simulink model "ModelDemopalooza"  (R2022b)
settings: Solver=FixedStepDiscrete  StartTime=0.0  StopTime=1  RelTol=1e-3  EnableMultiTasking=on
InitFcn:
  | % Initialize model
  | run(['ModelInit.m']);
  | 
  | % load library data
  | GainLibrary_data;
StartFcn:
  | % make sure all the simulated RTC requests are found
  | %RTC_SIM_OBJ.ValidateREQs();
model workspace (MAT data in the model file):
  PreampVolumeTable_Idx = Simulink.Signal
  PreampVolumeTable_Idx.DataType = 'auto'
  PreampVolumeTable_Idx.Dimensions = -1
  PreampVolumeTable_Idx.DimensionsMode = 'auto'
  PreampVolumeTable_Idx.Complexity = 'auto'
  PreampVolumeTable_Idx.SampleTime = -1
  PreampVolumeTable_Idx.SamplingMode = 'auto'
  PreampVolumeTable_Idx.InitialValue = 'uint8([0 255 255 255 255 255])'
  Range = Simulink.Signal
  Range.DataType = 'auto'
  Range.Dimensions = -1
  Range.DimensionsMode = 'auto'
  Range.Complexity = 'auto'
  Range.SampleTime = -1
  Range.SamplingMode = 'auto'
  Table_Idx = Simulink.Signal
  Table_Idx.DataType = 'auto'
  Table_Idx.Dimensions = -1
  Table_Idx.DimensionsMode = 'auto'
  Table_Idx.Complexity = 'auto'
  Table_Idx.SampleTime = -1
  Table_Idx.SamplingMode = 'auto'
undefined symbols (not defined in the file): Config, Ifir, IFIR, MedusaConfig, MuteRamper, MuteRamperBtc, numAudioIn, preAmp, Row, sys_defs, VLSConfig
libraries: FeaturePath x22, TuneVar x17, RTC x9, MedusaDelays x9, dspindex x5, TOP x5, SampleRateConverter x4, EdgePorts x2, PooliirLib x2, MedusaCaeEnable x2, FIREven x2, VLSGains x2
(part 1 of 4)
settings Model: Creator=kl13806  LastModifiedBy=sc48041
settings SolverCC: AlgebraicLoopSolver=TrustRegion  AutoInsertRateTranBlk=on
settings OptimizationCC: DefaultParameterBehavior=Inlined  DefaultUnderspecifiedDataType=single  ZeroExternalMemoryAtStartup=off  ZeroInternalMemoryAtStartup=off  MaxStackSize=2048  DifferentSizesBufferReuse=on  EfficientTunableParamExpr=on
settings DebuggingCC: InheritedTsInSrcMsg=none  MultiTaskDSMMsg=none  MultiTaskRateTransMsg=warning  ParameterPrecisionLossMsg=none  ParameterTunabilityLossMsg=error  UnconnectedInputMsg=warning  UnconnectedOutputMsg=warning  UnconnectedLineMsg=warning  BusObjectLabelMismatch=none  UnknownTsInhSupMsg=none  SFUnexpectedBacktrackingDiag=warning  SFNoUnconditionalDefaultTransitionDiag=warning  SFExecutionAtInitializationDiag=none  SFMachineParentedDataDiag=warning  ArithmeticOperatorsInVariantConditions=warning
settings HardwareCC: ProdBitPerDouble=32  ProdBitPerPointer=32  ProdBitPerSizeT=32  ProdBitPerPtrDiffT=32  ProdLargestAtomicInteger=Long  ProdLargestAtomicFloat=Double  ProdWordSize=32  ProdHWDeviceType=Qualcomm->Hexagon  TargetBitPerPointer=64  TargetBitPerSizeT=64  TargetBitPerPtrDiffT=64  TargetLargestAtomicInteger=Integer  TargetLongLongMode=on  TargetIntDivRoundTo=Zero  TargetEndianess=LittleEndian  TargetWordSize=64  TargetHWDeviceType=MATLAB Host  ProdEqTarget=off
settings ModelReferenceCC: EnableRefExpFcnMdlSchedulingChecks=on
settings SFSimCC: SimUseLocalCustomCode=off  MATLABDynamicMemAlloc=off  CustomCodeUndefinedFunction=UseInterfaceOnly
settings RTWCC: Description=Embedded Coder (host-based shared library target)  SystemTargetFile=ert_shrlib.tlc  GenCodeOnly=on  TemplateMakefile=ert_default_tmf  GenerateReport=on  RetainRTWFile=on  RTWUseLocalCustomCode=off  BuildConfiguration=Faster Runs  IncludeHyperlinkInReport=on  LaunchReport=on  GenerateTraceInfo=on  GenerateTraceReport=on  GenerateTraceReportSl=on  GenerateTraceReportSf=on  GenerateTraceReportEml=on  GenerateCodeMetricsReport=on  GenerateCodeReplacementReport=on
settings CodeAppCC: ForceParamTrailComments=on  IgnoreCustomStorageClasses=off  MaxIdLength=61  OperatorAnnotations=on  SimulinkDataObjDesc=on  SFDataObjDesc=on  MATLABFcnDesc=on  InsertBlockDesc=on  StateflowObjectComments=on  MATLABSourceComments=on
settings STFCustomTargetCC: TargetLangStandard=C99 (ISO)  CodeReplacementLibrary=Qualcomm Hexagon DSP code replacement library  ParMdlRefBuildCompliant=on  CompOptLevelCompliant=on  CombineOutputUpdateFcns=on  ERTCustomFileBanners=on  SupportNonFinite=off  SupportContinuousTime=off  SupportNonInlinedSFcns=off  RemoveResetFunc=on  SupportVariableSizeSignals=on  MATLABClassNameForMDSCustomization=Simulink.SoftwareTarget.ERTCustomization  ModelStepFunctionPrototypeControlCompliant=on  UseToolchainInfoCompliant=on  SystemTargetFile=ert_shrlib.tlc
settings ERTTargetCC: TargetLangStandard=C99 (ISO)  CodeReplacementLibrary=Qualcomm Hexagon DSP code replacement library  MultiwordLength=2048  ConcurrentExecutionCompliant=off  SupportNonFinite=off  SupportVariableSizeSignals=on  CPPClassGenCompliant=off  InlinedParameterPlacement=NonHierarchical  ERTCustomFileTemplate=example_file_process.tlc  IndentStyle=Allman  IndentSize=4
settings ConfigComp: CovMetricSettings=dw  CovSaveCumulativeToWorkspaceVar=on  CovSaveSingleToWorkspaceVar=on  CovExternalEMLEnable=off

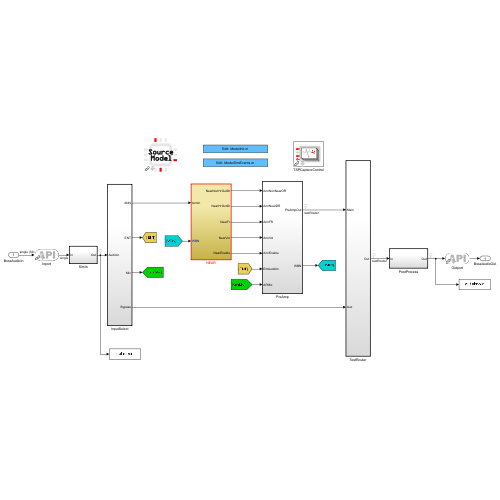
[thumbnail: Simulink's stored preview of the top-level diagram]
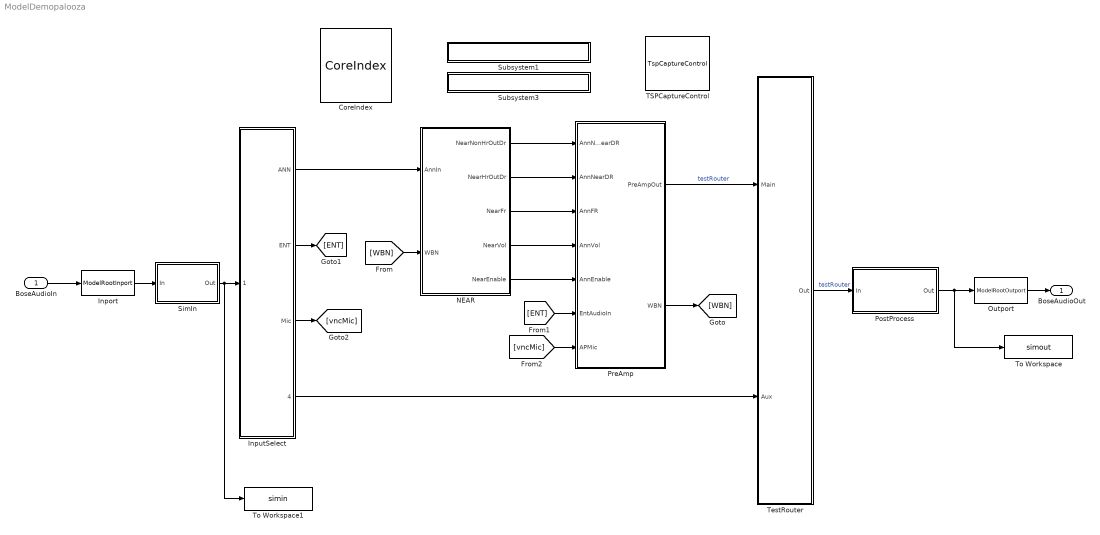
== system ModelDemopalooza ==
  BoseAudioIn : Inport  OutDataTypeStr=single  PortDimensions=[sys_defs.frameSize numAudioIn]  SampleTime=1/sys_defs.Fs * sys_defs.frameSize
  CoreIndex : FeaturePath/CoreIndex  Role=Source Model  CoreIndex=8  Config=[]  AddressingMode=Directly include core number in message identifiers (i.e. simple and static)  CrossCoreApi=None  CrossCoreAllocation=None  CrossCoreSampleTime=-1  BasePeriod=[]  TriggerInit=[-15 -776 80 -679]
      settings: SourceProductName=Bose Talaria
  Inport : EdgePorts/ModelRootInport  Config=ModelRootIn
      settings: SourceProductName=Bose Talaria
  InputSelect : Subsystem  TreatAsAtomicUnit=on
      settings: RTWSystemCode=Nonreusable function
  NEAR : Subsystem  TreatAsAtomicUnit=on
  Outport : EdgePorts/ModelRootOutport  Config=ModelRootOut
      settings: SourceProductName=Bose Talaria
  PostProcess : Subsystem  TreatAsAtomicUnit=on
  PreAmp : Subsystem  TreatAsAtomicUnit=on
  SimIn : Subsystem  TreatAsAtomicUnit=on
  Subsystem1 : Subsystem  mask{filename=Init.m}
      settings: OpenFcn=edit([ ModelRootName() get(gcbh,'filename') ]);
      mask Display: disp(['Edit: ' ModelRootName() get(gcbh,'filename')]);
  Subsystem3 : Subsystem  mask{filename=SimEvents.m}
      settings: OpenFcn=edit([ ModelRootName() get(gcbh,'filename') ]);
      mask Display: disp(['Edit: ' ModelRootName() get(gcbh,'filename')]);
  TSPCaptureControl : TSP/TspCaptureControl  TriggerInit=[415 -766 500 -694]
      settings: SourceProductName=Bose Talaria
  TestRouter : Subsystem  TreatAsAtomicUnit=on
  To Workspace : ToWorkspace  VariableName=simout  SaveFormat=Timeseries  SampleTime=-1
  To Workspace1 : ToWorkspace  VariableName=simin  SaveFormat=Timeseries  SampleTime=-1
  BoseAudioOut : Outport  VectorParamsAs1DForOutWhenUnconnected=off
  wires:
  SimIn/1(Out) -> To Workspace1/1, InputSelect/1(AudioIn)
  BoseAudioIn/1 -> Inport/1
  Inport/1 -> SimIn/1(In)
  Outport/1 -> BoseAudioOut/1
  InputSelect/1(ANN) -> NEAR/1(AnnIn)
  [WBN] -> NEAR/2(WBN)
  NEAR/5(NearEnable) -> PreAmp/5(AnnEnable)
  NEAR/4(NearVol) -> PreAmp/4(AnnVol)
  NEAR/3(NearFr) -> PreAmp/3(AnnFR)
  PreAmp/2(WBN) -> [WBN]
  NEAR/1(NearNonHrOutDr) -> PreAmp/1(AnnNonNearDR)
  NEAR/2(NearHrOutDr) -> PreAmp/2(AnnNearDR)
  InputSelect/2(ENT) -> [ENT]
  [ENT] -> PreAmp/6(EntAudioIn)
  InputSelect/3(Mic) -> [vncMic]
  [vncMic] -> PreAmp/7(APMic)
  PreAmp/1(PreAmpOut) -> TestRouter/1(Main)  "testRouter"
  TestRouter/1(Out) -> PostProcess/1(In)  "testRouter"
  PostProcess/1(Out) -> To Workspace/1, Outport/1
  InputSelect/4(Bypass) -> TestRouter/2(Aux)

== system ModelDemopalooza/InputSelect ==
  AudioIn : Inport
  FeaturePath : FeaturePath/FeaturePath  FeatureName=InputSelect  IsGroup=on  GroupNumber=0  IsModule=on  TriggerInit=[105 216 220 329]
      settings: SourceProductName=Bose Talaria
  Partition : FeaturePath/Partition  PartitionNumber=0  TriggerInit=[250 241 295 309]
      settings: SourceProductName=Bose Talaria
  Reset : Subsystem  Commented=on
  Variable Selector1 : dspindex/Variable Selector  NumInputs=1  rowsOrCols=Columns  IdxMode=Fixed  Elements=entMap  ZerOneIdxMode=One-based  errmode=Clip Index  FillMode=on  FillValues=0
  Variable Selector2 : dspindex/Variable Selector  NumInputs=1  rowsOrCols=Columns  IdxMode=Fixed  Elements=annMap  ZerOneIdxMode=One-based  errmode=Clip Index  FillMode=on  FillValues=0
  Variable Selector3 : dspindex/Variable Selector  NumInputs=1  rowsOrCols=Columns  IdxMode=Fixed  Elements=vncMic  ZerOneIdxMode=One-based  errmode=Clip Index  FillMode=on  FillValues=0
  router : Router/Router  nInRouterMask=inputSelectChanIn  nOutRouterMask=inputSelectChanOut  outputMapDefaultRouterMask=inputSelectOutputMap
  ANN : Outport
  ENT : Outport  Port=2  VectorParamsAs1DForOutWhenUnconnected=off
  Mic : Outport  Port=3
  Bypass : Outport  Port=4  VectorParamsAs1DForOutWhenUnconnected=off
  wires:
  Variable Selector1/1 -> ENT/1
  AudioIn/1 -> Bypass/1, router/1
  router/1 -> Variable Selector3/1, Variable Selector2/1, Variable Selector1/1
  Variable Selector2/1 -> ANN/1
  Variable Selector3/1 -> Mic/1

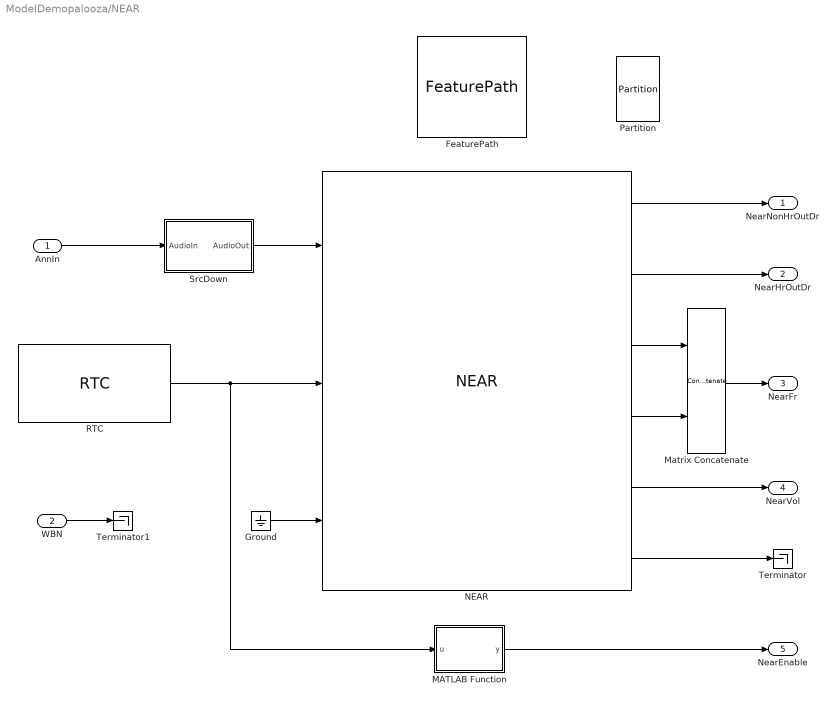
== system ModelDemopalooza/NEAR ==
  AnnIn : Inport
  WBN : Inport  Port=2
  FeaturePath : FeaturePath/FeaturePath  FeatureName=Near  IsGroup=on  GroupNumber=1  IsModule=on  TriggerInit=[15 -306 130 -199]
      settings: SourceProductName=Bose Talaria
  Ground : Ground
  MATLAB Function : MATLAB Function  TreatAsAtomicUnit=on
  Matrix Concatenate : Concatenate  Mode=Multidimensional array  ConcatenateDimension=2
  NEAR : Near1p1Ann/NEAR  near=near
  Partition : FeaturePath/Partition  PartitionNumber=0  TriggerInit=[225 -284 270 -216]
      settings: SourceProductName=Bose Talaria
  RTC : RTC/RTC  REQ_Priority=RTC_Mask.NormalPriority  RequestAtInit=off  EnableRequest=off  REQElemName1=Enable  REQElemType1=uint32  REQElemWidth1=1  REQElemInitial1=[0]  REQElemType2=uint32  REQElemWidth2=1  REQElemInitial2=[]  REQElemType3=uint32  REQElemWidth3=1  REQElemInitial3=[]  REQElemType4=uint32  REQElemWidth4=1  REQElemInitial4=[]  REQElemType5=uint32  REQElemWidth5=1  REQElemInitial5=[]  REQElemType6=uint32  REQElemWidth6=1  REQElemInitial6=[]  REQElemType7=uint32  REQElemWidth7=1  REQElemInitial7=[]  REQElemType8=uint32  REQElemWidth8=1  REQElemInitial8=[]  REQElemType9=uint32  REQElemWidth9=1  REQElemInitial9=[]  REQElemType10=uint32  REQElemWidth10=1  REQElemInitial10=[]  EnableResponse=on  EnableRSP_StatusIn=off  RSPElemType1=uint32  RSPElemWidth1=1  RSPElemType2=uint32  RSPElemWidth2=1  RSPElemType3=uint32  RSPElemWidth3=1  RSPElemType4=uint32  RSPElemWidth4=1  RSPElemType5=uint32  RSPElemWidth5=1  RSPElemType6=uint32  RSPElemWidth6=1  RSPElemType7=uint32  RSPElemWidth7=1  RSPElemType8=uint32  RSPElemWidth8=1  RSPElemType9=uint32  RSPElemWidth9=1  RSPElemType10=uint32  RSPElemWidth10=1  EnableNotification=off  EnableNTF_PrepTrig=off  NTFElemType1=uint32  NTFElemWidth1=1  NTFElemType2=uint32  NTFElemWidth2=1  NTFElemType3=uint32  NTFElemWidth3=1  NTFElemType4=uint32  NTFElemWidth4=1  NTFElemType5=uint32  NTFElemWidth5=1  NTFElemType6=uint32  NTFElemWidth6=1  NTFElemType7=uint32  NTFElemWidth7=1  NTFElemType8=uint32  NTFElemWidth8=1  NTFElemType9=uint32  NTFElemWidth9=1  NTFElemType10=uint32  NTFElemWidth10=1  MaskMessageName=Enable
      settings: SourceProductName=Bose Talaria
  SrcDown : Subsystem  TreatAsAtomicUnit=on
      settings: RTWSystemCode=Nonreusable function
  Terminator : Terminator
  Terminator1 : Terminator
  NearNonHrOutDr : Outport
  NearHrOutDr : Outport  Port=2
  NearFr : Outport  Port=3
  NearVol : Outport  Port=4
  NearEnable : Outport  Port=5
  wires:
  NEAR/1 -> NearNonHrOutDr/1
  AnnIn/1 -> SrcDown/1(AudioIn)
  NEAR/2 -> NearHrOutDr/1
  NEAR/3 -> Matrix Concatenate/1
  NEAR/4 -> Matrix Concatenate/2
  Matrix Concatenate/1 -> NearFr/1
  NEAR/5 -> NearVol/1
  NEAR/6 -> Terminator/1
  RTC/1 -> NEAR/2, MATLAB Function/1(u)
  MATLAB Function/1(y) -> NearEnable/1
  SrcDown/1(AudioOut) -> NEAR/1
  Ground/1 -> NEAR/3
  WBN/1 -> Terminator1/1

== system ModelDemopalooza/PostProcess ==
  In : Inport
  FeaturePath : FeaturePath/FeaturePath  FeatureName=PostProcess  IsGroup=on  GroupNumber=3  IsModule=on  TriggerInit=[85 -186 200 -79]
      settings: SourceProductName=Bose Talaria
  Partition : FeaturePath/Partition  PartitionNumber=0  TriggerInit=[225 -164 270 -96]
      settings: SourceProductName=Bose Talaria
  PostProcess : Subsystem  TreatAsAtomicUnit=on
      settings: RTWSystemCode=Nonreusable function  RTWFcnNameOpts=Use subsystem name  RTWFileNameOpts=Use subsystem name  FunctionWithSeparateData=on
  Reset : Subsystem  Commented=on
  Out : Outport  VectorParamsAs1DForOutWhenUnconnected=off
  wires:
  In/1 -> PostProcess/1(In)
  PostProcess/1(Out) -> Out/1

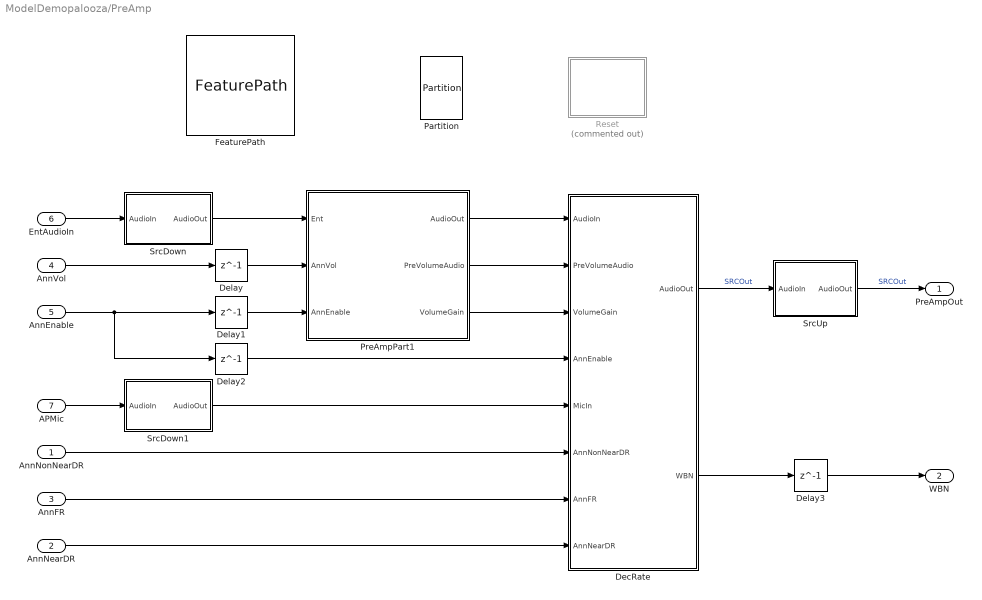
== system ModelDemopalooza/PreAmp ==
  AnnNonNearDR : Inport
  AnnNearDR : Inport  Port=2
  AnnFR : Inport  Port=3
  AnnVol : Inport  Port=4
  AnnEnable : Inport  Port=5
  EntAudioIn : Inport  Port=6
  APMic : Inport  Port=7
  DecRate : Subsystem
  Delay{,1..3} (4 alike) : Delay  DelayLength=1
  FeaturePath : FeaturePath/FeaturePath  FeatureName=PreAmp  IsGroup=on  GroupNumber=2  IsModule=on  TriggerInit=[-135 -246 -20 -139]
      settings: SourceProductName=Bose Talaria
  Partition : FeaturePath/Partition  PartitionNumber=0  TriggerInit=[115 -224 160 -156]
      settings: SourceProductName=Bose Talaria
  PreAmpPart1 : Subsystem  TreatAsAtomicUnit=on
      settings: RTWSystemCode=Nonreusable function
  Reset : Subsystem  Commented=on
  SrcDown : Subsystem  TreatAsAtomicUnit=on
      settings: RTWSystemCode=Nonreusable function
  SrcDown1 : Subsystem  TreatAsAtomicUnit=on
      settings: RTWSystemCode=Nonreusable function
  SrcUp : Subsystem  TreatAsAtomicUnit=on
      settings: RTWSystemCode=Nonreusable function
  PreAmpOut : Outport  VectorParamsAs1DForOutWhenUnconnected=off
  WBN : Outport  Port=2
  wires:
  EntAudioIn/1 -> SrcDown/1(AudioIn)
  DecRate/1(AudioOut) -> SrcUp/1(AudioIn)  "SRCOut"
  SrcUp/1(AudioOut) -> PreAmpOut/1  "SRCOut"
  Delay3/1 -> WBN/1
  SrcDown/1(AudioOut) -> PreAmpPart1/1(Ent)
  AnnVol/1 -> Delay/1
  AnnEnable/1 -> Delay2/1, Delay1/1
  Delay/1 -> PreAmpPart1/2(AnnVol)
  Delay1/1 -> PreAmpPart1/3(AnnEnable)
  AnnNonNearDR/1 -> DecRate/6(AnnNonNearDR)
  AnnNearDR/1 -> DecRate/8(AnnNearDR)
  AnnFR/1 -> DecRate/7(AnnFR)
  APMic/1 -> SrcDown1/1(AudioIn)
  PreAmpPart1/1(AudioOut) -> DecRate/1(AudioIn)
  PreAmpPart1/2(PreVolumeAudio) -> DecRate/2(PreVolumeAudio)
  PreAmpPart1/3(VolumeGain) -> DecRate/3(VolumeGain)
  Delay2/1 -> DecRate/4(AnnEnable)
  DecRate/2(WBN) -> Delay3/1
  SrcDown1/1(AudioOut) -> DecRate/5(MicIn)

== system ModelDemopalooza/SimIn ==
  In : Inport  OutDataTypeStr=single  SampleTime=1/sys_defs.Fs * sys_defs.frameSize
  Colored Noise : dspsrcs4/Colored Noise  Commented=on  Color=pink  InverseFrequencyPower=1  BoundedOutput=on  NumChannels=2  OutputDataType=single  SamplesPerFrame=32  SampleTime=1/48000  RandomStream=mt19937ar with seed  Seed=67  SimulateUsing=Interpreted execution
  Sine Wave : dspsrcs4/Sine Wave  Amplitude=[0.1*ones(1,numAudioIn)]  Frequency=[150 225 200 275 325]  Phase=zeros(1,numAudioIn)  SampleMode=Discrete  OutComplex=Real  CompMethod=Trigonometric fcn  TableSize=Speed  SampleTime=1/sys_defs.Fs  SamplesPerFrame=sys_defs.frameSize  ResetState=Restart at time zero  OutputFrames=off  dataType=single  wordLen=16  udDataType=sfix(16)  fracBitsMode=Best precision  numFracBits=15  OutDataTypeStr=single  LastOutDataTypeStr=single
  Variant Source : VariantSource  VariantControlMode=sim codegen switching  ShowConditionOnBlock=on
  Out : Outport  VectorParamsAs1DForOutWhenUnconnected=off
  wires:
  In/1 -> Variant Source/2
  Variant Source/1 -> Out/1
  Sine Wave/1 -> Variant Source/1

== system ModelDemopalooza/Subsystem1 ==

== system ModelDemopalooza/Subsystem3 ==

== system ModelDemopalooza/TestRouter ==
  Main : Inport
  Aux : Inport  Port=2
  ASDRouter : ASDRouter/ASDRouter  frameSize=sys_defs.frameSize  nChanOut=sys_defs.nAudioOut  mainSelect=main_select_test  numMainCh=num_main_chs  mainGain=main_gain_test  enableAux=enableAuxTestFlag  numAux=numAuxTestChannels  auxGain=aux_gain_test
  FeaturePath : FeaturePath/FeaturePath  FeatureName=TestRouter  IsGroup=on  GroupNumber=5  IsModule=off  TriggerInit=[290 -166 405 -59]
      settings: SourceProductName=Bose Talaria
  Matrix Concatenate : Concatenate  Mode=Multidimensional array  ConcatenateDimension=2
  Partition : FeaturePath/Partition  PartitionNumber=0  TriggerInit=[470 -149 515 -81]
      settings: SourceProductName=Bose Talaria
  TuneTOP : TuneVar/TuneTOP  TriggerInit=[175 117 345 173]  TopName=AuxSelect  TuneName=AuxSelect  DataType=int32  TunabilityNumber=1  MinValue=[]  MaxValue=[]  BankNumber=0  PreOverlay=false  PostOverlay=false  UseSameName=on  MaskValue=aux_select_test
      settings: SourceProductName=Bose Talaria
  Out : Outport
  wires:
  ASDRouter/1 -> Out/1
  TuneTOP/1 -> ASDRouter/2
  Matrix Concatenate/1 -> ASDRouter/1
  Main/1 -> Matrix Concatenate/1
  Aux/1 -> Matrix Concatenate/2

== system ModelDemopalooza/InputSelect/Reset ==
  MATLAB Function : MATLAB Function  TreatAsAtomicUnit=on
  RTC : RTC/RTC  REQ_Priority=RTC_Mask.NormalPriority  RequestAtInit=off  EnableRequest=on  REQElemType1=uint32  REQElemWidth1=1  REQElemInitial1=[]  REQElemType2=uint32  REQElemWidth2=1  REQElemInitial2=[]  REQElemType3=uint32  REQElemWidth3=1  REQElemInitial3=[]  REQElemType4=uint32  REQElemWidth4=1  REQElemInitial4=[]  REQElemType5=uint32  REQElemWidth5=1  REQElemInitial5=[]  REQElemType6=uint32  REQElemWidth6=1  REQElemInitial6=[]  REQElemType7=uint32  REQElemWidth7=1  REQElemInitial7=[]  REQElemType8=uint32  REQElemWidth8=1  REQElemInitial8=[]  REQElemType9=uint32  REQElemWidth9=1  REQElemInitial9=[]  REQElemType10=uint32  REQElemWidth10=1  REQElemInitial10=[]  EnableResponse=on  EnableRSP_StatusIn=off  RSPElemType1=uint32  RSPElemWidth1=1  RSPElemType2=uint32  RSPElemWidth2=1  RSPElemType3=uint32  RSPElemWidth3=1  RSPElemType4=uint32  RSPElemWidth4=1  RSPElemType5=uint32  RSPElemWidth5=1  RSPElemType6=uint32  RSPElemWidth6=1  RSPElemType7=uint32  RSPElemWidth7=1  RSPElemType8=uint32  RSPElemWidth8=1  RSPElemType9=uint32  RSPElemWidth9=1  RSPElemType10=uint32  RSPElemWidth10=1  EnableNotification=off  EnableNTF_PrepTrig=off  NTFElemType1=uint32  NTFElemWidth1=1  NTFElemType2=uint32  NTFElemWidth2=1  NTFElemType3=uint32  NTFElemWidth3=1  NTFElemType4=uint32  NTFElemWidth4=1  NTFElemType5=uint32  NTFElemWidth5=1  NTFElemType6=uint32  NTFElemWidth6=1  NTFElemType7=uint32  NTFElemWidth7=1  NTFElemType8=uint32  NTFElemWidth8=1  NTFElemType9=uint32  NTFElemWidth9=1  NTFElemType10=uint32  NTFElemWidth10=1  MaskMessageName=Reset
      settings: SourceProductName=Bose Talaria
  wires:
  RTC/1 -> MATLAB Function/Trigger

== system ModelDemopalooza/NEAR/SrcDown ==
  AudioIn : Inport
  Frame Conversion1 : FrameConversion  OutFrame=Sample-based
  Frame Conversion2 : FrameConversion
  SampleRateConverter : SampleRateConverter/SampleRateConverter  UPFACTOR=12  DOWNFACTOR=13  OUTFRAME_SIZE=-1  RATE_SELECTOR=Input Sample Rate  FS=48000  FPASSBAND=16500  FHEARING=19000  PASSBAND_RIPPLE=60  STOPBAND_ATTENUATION=60
  AudioOut : Outport
  wires:
  SampleRateConverter/1 -> Frame Conversion1/1
  AudioIn/1 -> Frame Conversion2/1
  Frame Conversion1/1 -> AudioOut/1
  Frame Conversion2/1 -> SampleRateConverter/1

== system ModelDemopalooza/PostProcess/PostProcess ==
  In : Inport
  EnergyLimiter : Subsystem
  Goto Tag Visibility : GotoTagVisibility  GotoTag=EntLimiterSoftclipParamSet
  Goto Tag Visibility1 : GotoTagVisibility  GotoTag=EntLimiterSoftclipDisableMsg
  Limiter : Subsystem
  Mute : Subsystem
  OutputEQ : Subsystem
  RTC : RTC/RTC  Description=|  REQ_Priority=RTC_Mask.NormalPriority  RequestAtInit=off  EnableRequest=off  REQElemName1=paramSet  REQElemType1=uint32  REQElemWidth1=1  REQElemInitial1=1  REQElemType2=uint32  REQElemWidth2=1  REQElemInitial2=[]  REQElemType3=uint32  REQElemWidth3=1  REQElemInitial3=[]  REQElemType4=uint32  REQElemWidth4=1  REQElemInitial4=[]  REQElemType5=uint32  REQElemWidth5=1  REQElemInitial5=[]  REQElemType6=uint32  REQElemWidth6=1  REQElemInitial6=[]  REQElemType7=uint32  REQElemWidth7=1  REQElemInitial7=[]  REQElemType8=uint32  REQElemWidth8=1  REQElemInitial8=[]  REQElemType9=uint32  REQElemWidth9=1  REQElemInitial9=[]  REQElemType10=uint32  REQElemWidth10=1  REQElemInitial10=[]  EnableResponse=on  EnableRSP_StatusIn=off  RSPElemName1=paramSet  RSPElemType1=uint32  RSPElemWidth1=1  RSPElemType2=uint32  RSPElemWidth2=1  RSPElemType3=uint32  RSPElemWidth3=1  RSPElemType4=uint32  RSPElemWidth4=1  RSPElemType5=uint32  RSPElemWidth5=1  RSPElemType6=uint32  RSPElemWidth6=1  RSPElemType7=uint32  RSPElemWidth7=1  RSPElemType8=uint32  RSPElemWidth8=1  RSPElemType9=uint32  RSPElemWidth9=1  RSPElemType10=uint32  RSPElemWidth10=1  EnableNotification=off  EnableNTF_PrepTrig=off  NTFElemType1=uint32  NTFElemWidth1=1  NTFElemType2=uint32  NTFElemWidth2=1  NTFElemType3=uint32  NTFElemWidth3=1  NTFElemType4=uint32  NTFElemWidth4=1  NTFElemType5=uint32  NTFElemWidth5=1  NTFElemType6=uint32  NTFElemWidth6=1  NTFElemType7=uint32  NTFElemWidth7=1  NTFElemType8=uint32  NTFElemWidth8=1  NTFElemType9=uint32  NTFElemWidth9=1  NTFElemType10=uint32  NTFElemWidth10=1  MaskMessageName=LimiterSoftclipParamSet
      | Choose parameter set for limiter and soft clipper.
      | 1: normal set
      | 2: used in start-stop situation
      settings: SourceProductName=Bose Talaria
  RTC1 : RTC/RTC  REQ_Priority=RTC_Mask.NormalPriority  RequestAtInit=off  EnableRequest=off  REQElemName1=disableMsg  REQElemType1=uint32  REQElemWidth1=1  REQElemInitial1=0  REQElemType2=uint32  REQElemWidth2=1  REQElemInitial2=[]  REQElemType3=uint32  REQElemWidth3=1  REQElemInitial3=[]  REQElemType4=uint32  REQElemWidth4=1  REQElemInitial4=[]  REQElemType5=uint32  REQElemWidth5=1  REQElemInitial5=[]  REQElemType6=uint32  REQElemWidth6=1  REQElemInitial6=[]  REQElemType7=uint32  REQElemWidth7=1  REQElemInitial7=[]  REQElemType8=uint32  REQElemWidth8=1  REQElemInitial8=[]  REQElemType9=uint32  REQElemWidth9=1  REQElemInitial9=[]  REQElemType10=uint32  REQElemWidth10=1  REQElemInitial10=[]  EnableResponse=on  EnableRSP_StatusIn=off  RSPElemName1=disableMsg  RSPElemType1=uint32  RSPElemWidth1=1  RSPElemType2=uint32  RSPElemWidth2=1  RSPElemType3=uint32  RSPElemWidth3=1  RSPElemType4=uint32  RSPElemWidth4=1  RSPElemType5=uint32  RSPElemWidth5=1  RSPElemType6=uint32  RSPElemWidth6=1  RSPElemType7=uint32  RSPElemWidth7=1  RSPElemType8=uint32  RSPElemWidth8=1  RSPElemType9=uint32  RSPElemWidth9=1  RSPElemType10=uint32  RSPElemWidth10=1  EnableNotification=off  EnableNTF_PrepTrig=off  NTFElemType1=uint32  NTFElemWidth1=1  NTFElemType2=uint32  NTFElemWidth2=1  NTFElemType3=uint32  NTFElemWidth3=1  NTFElemType4=uint32  NTFElemWidth4=1  NTFElemType5=uint32  NTFElemWidth5=1  NTFElemType6=uint32  NTFElemWidth6=1  NTFElemType7=uint32  NTFElemWidth7=1  NTFElemType8=uint32  NTFElemWidth8=1  NTFElemType9=uint32  NTFElemWidth9=1  NTFElemType10=uint32  NTFElemWidth10=1  MaskMessageName=LimiterSoftclipDisable
      settings: SourceProductName=Bose Talaria
  Soft Clipper : Subsystem
  Out : Outport  VectorParamsAs1DForOutWhenUnconnected=off
  tag scope: EntLimiterSoftclipDisableMsg=scoped, EntLimiterSoftclipParamSet=scoped
  wires:
  Mute/1(Out1) -> Limiter/1(In1)
  Limiter/1(Out1) -> OutputEQ/1(In1)
  In/1 -> Mute/1(In1)
  OutputEQ/1(Out1) -> EnergyLimiter/1(In1)
  EnergyLimiter/1(Out1) -> Soft Clipper/1(In1)
  RTC1/1 -> RTC1/1, [EntLimiterSoftclipDisableMsg]
  RTC/1 -> RTC/1, [EntLimiterSoftclipParamSet]
  Soft Clipper/1(Out1) -> Out/1

== system ModelDemopalooza/PostProcess/Reset ==
  MATLAB Function : MATLAB Function  TreatAsAtomicUnit=on
  RTC : RTC/RTC  REQ_Priority=RTC_Mask.NormalPriority  RequestAtInit=off  EnableRequest=on  REQElemType1=uint32  REQElemWidth1=1  REQElemInitial1=[]  REQElemType2=uint32  REQElemWidth2=1  REQElemInitial2=[]  REQElemType3=uint32  REQElemWidth3=1  REQElemInitial3=[]  REQElemType4=uint32  REQElemWidth4=1  REQElemInitial4=[]  REQElemType5=uint32  REQElemWidth5=1  REQElemInitial5=[]  REQElemType6=uint32  REQElemWidth6=1  REQElemInitial6=[]  REQElemType7=uint32  REQElemWidth7=1  REQElemInitial7=[]  REQElemType8=uint32  REQElemWidth8=1  REQElemInitial8=[]  REQElemType9=uint32  REQElemWidth9=1  REQElemInitial9=[]  REQElemType10=uint32  REQElemWidth10=1  REQElemInitial10=[]  EnableResponse=on  EnableRSP_StatusIn=off  RSPElemType1=uint32  RSPElemWidth1=1  RSPElemType2=uint32  RSPElemWidth2=1  RSPElemType3=uint32  RSPElemWidth3=1  RSPElemType4=uint32  RSPElemWidth4=1  RSPElemType5=uint32  RSPElemWidth5=1  RSPElemType6=uint32  RSPElemWidth6=1  RSPElemType7=uint32  RSPElemWidth7=1  RSPElemType8=uint32  RSPElemWidth8=1  RSPElemType9=uint32  RSPElemWidth9=1  RSPElemType10=uint32  RSPElemWidth10=1  EnableNotification=off  EnableNTF_PrepTrig=off  NTFElemType1=uint32  NTFElemWidth1=1  NTFElemType2=uint32  NTFElemWidth2=1  NTFElemType3=uint32  NTFElemWidth3=1  NTFElemType4=uint32  NTFElemWidth4=1  NTFElemType5=uint32  NTFElemWidth5=1  NTFElemType6=uint32  NTFElemWidth6=1  NTFElemType7=uint32  NTFElemWidth7=1  NTFElemType8=uint32  NTFElemWidth8=1  NTFElemType9=uint32  NTFElemWidth9=1  NTFElemType10=uint32  NTFElemWidth10=1  MaskMessageName=Reset
      settings: SourceProductName=Bose Talaria
  wires:
  RTC/1 -> MATLAB Function/Trigger

== system ModelDemopalooza/PreAmp/DecRate ==
  AudioIn : Inport
  PreVolumeAudio : Inport  Port=2
  VolumeGain : Inport  Port=3
  AnnEnable : Inport  Port=4
  MicIn : Inport  Port=5
  AnnNonNearDR : Inport  Port=6
  AnnFR : Inport  Port=7
  AnnNearDR : Inport  Port=8
  AudioPilot35 : Subsystem
  Constant : Constant  Value=0
  Delay : Delay  DelayLength=1
  Medusa5H1 : Subsystem
  AudioOut : Outport
  WBN : Outport  Port=2
  wires:
  Medusa5H1/1(AudioOut) -> AudioOut/1
  PreVolumeAudio/1 -> AudioPilot35/3(PreVolumeAudio)
  MicIn/1 -> AudioPilot35/2(Mic)
  AudioPilot35/2(WBNoisedbspl) -> Delay/1
  Delay/1 -> WBN/1
  VolumeGain/1 -> AudioPilot35/4(VolumeGain)
  Medusa5H1/2(LFRef) -> AudioPilot35/5(LFRef)
  Medusa5H1/3(HFRef) -> AudioPilot35/6(HFRefLPF)
  Constant/1 -> AudioPilot35/7(AnnTrigger)
  AnnEnable/1 -> Medusa5H1/5(AnnEnable)
  AnnNonNearDR/1 -> Medusa5H1/2(AnnNonHeadrestDR)
  AnnNearDR/1 -> Medusa5H1/3(AnnHeadrestDR)
  AnnFR/1 -> Medusa5H1/4(AnnFR)
  AudioIn/1 -> AudioPilot35/1(MusicIn)
  AudioPilot35/1(MusicOut) -> Medusa5H1/1(AudioIn)

== system ModelDemopalooza/PreAmp/PreAmpPart1 ==
  Ent : Inport
  AnnVol : Inport  Port=2
  AnnEnable : Inport  Port=3
  Bass : ToneBtc/Tone  FeatureName=Bass  Config=[]  TriggerInit=[215 80 320 140]
      settings: SourceProductName=Bose Blocklib
  Delay : Delay  DelayLength=1
  Midrange : MidrangeBtc/Midrange  FeatureName=Midrange  Config=[]
      settings: SourceProductName=Bose Blocklib
  NEARPreAmp : PreAmpLib/PreAmp  Config=[preAmp]
  Treble : ToneBtc/Tone  FeatureName=Treble  Config=[]  TriggerInit=[395 80 500 140]
      settings: SourceProductName=Bose Blocklib
  Volume : VolumeBtc/Volume  FeatureName=Volume  Config=Volume  EnableGainOut=on  TriggerInit=[770 72 845 148]
      settings: SourceProductName=Bose Blocklib
  AudioOut : Outport
  PreVolumeAudio : Outport  Port=2
  VolumeGain : Outport  Port=3
  wires:
  Ent/1 -> NEARPreAmp/1
  Bass/1 -> Treble/1
  Treble/1 -> Midrange/1
  Midrange/1 -> PreVolumeAudio/1, Volume/1
  Volume/1 -> AudioOut/1
  Volume/2 -> Delay/1, VolumeGain/1
  NEARPreAmp/1 -> Bass/1
  Delay/1 -> NEARPreAmp/2
  AnnVol/1 -> NEARPreAmp/3
  AnnEnable/1 -> NEARPreAmp/4

== system ModelDemopalooza/PreAmp/Reset ==
  MATLAB Function : MATLAB Function  TreatAsAtomicUnit=on
  RTC : RTC/RTC  REQ_Priority=RTC_Mask.NormalPriority  RequestAtInit=off  EnableRequest=on  REQElemType1=uint32  REQElemWidth1=1  REQElemInitial1=[]  REQElemType2=uint32  REQElemWidth2=1  REQElemInitial2=[]  REQElemType3=uint32  REQElemWidth3=1  REQElemInitial3=[]  REQElemType4=uint32  REQElemWidth4=1  REQElemInitial4=[]  REQElemType5=uint32  REQElemWidth5=1  REQElemInitial5=[]  REQElemType6=uint32  REQElemWidth6=1  REQElemInitial6=[]  REQElemType7=uint32  REQElemWidth7=1  REQElemInitial7=[]  REQElemType8=uint32  REQElemWidth8=1  REQElemInitial8=[]  REQElemType9=uint32  REQElemWidth9=1  REQElemInitial9=[]  REQElemType10=uint32  REQElemWidth10=1  REQElemInitial10=[]  EnableResponse=on  EnableRSP_StatusIn=off  RSPElemType1=uint32  RSPElemWidth1=1  RSPElemType2=uint32  RSPElemWidth2=1  RSPElemType3=uint32  RSPElemWidth3=1  RSPElemType4=uint32  RSPElemWidth4=1  RSPElemType5=uint32  RSPElemWidth5=1  RSPElemType6=uint32  RSPElemWidth6=1  RSPElemType7=uint32  RSPElemWidth7=1  RSPElemType8=uint32  RSPElemWidth8=1  RSPElemType9=uint32  RSPElemWidth9=1  RSPElemType10=uint32  RSPElemWidth10=1  EnableNotification=off  EnableNTF_PrepTrig=off  NTFElemType1=uint32  NTFElemWidth1=1  NTFElemType2=uint32  NTFElemWidth2=1  NTFElemType3=uint32  NTFElemWidth3=1  NTFElemType4=uint32  NTFElemWidth4=1  NTFElemType5=uint32  NTFElemWidth5=1  NTFElemType6=uint32  NTFElemWidth6=1  NTFElemType7=uint32  NTFElemWidth7=1  NTFElemType8=uint32  NTFElemWidth8=1  NTFElemType9=uint32  NTFElemWidth9=1  NTFElemType10=uint32  NTFElemWidth10=1  MaskMessageName=Reset
      settings: SourceProductName=Bose Talaria
  wires:
  RTC/1 -> MATLAB Function/Trigger

== system ModelDemopalooza/PreAmp/SrcDown ==
  AudioIn : Inport
  Frame Conversion1 : FrameConversion  OutFrame=Sample-based
  Frame Conversion2 : FrameConversion
  SampleRateConverter : SampleRateConverter/SampleRateConverter  UPFACTOR=12  DOWNFACTOR=13  OUTFRAME_SIZE=-1  RATE_SELECTOR=Input Sample Rate  FS=48000  FPASSBAND=16500  FHEARING=19000  PASSBAND_RIPPLE=60  STOPBAND_ATTENUATION=60
  AudioOut : Outport
  wires:
  SampleRateConverter/1 -> Frame Conversion1/1
  AudioIn/1 -> Frame Conversion2/1
  Frame Conversion1/1 -> AudioOut/1
  Frame Conversion2/1 -> SampleRateConverter/1

== system ModelDemopalooza/PreAmp/SrcDown1 ==
  AudioIn : Inport
  Frame Conversion1 : FrameConversion  OutFrame=Sample-based
  Frame Conversion2 : FrameConversion
  SampleRateConverter : SampleRateConverter/SampleRateConverter  UPFACTOR=12  DOWNFACTOR=13  OUTFRAME_SIZE=-1  RATE_SELECTOR=Input Sample Rate  FS=48000  FPASSBAND=16500  FHEARING=19000  PASSBAND_RIPPLE=60  STOPBAND_ATTENUATION=60
  AudioOut : Outport
  wires:
  SampleRateConverter/1 -> Frame Conversion1/1
  AudioIn/1 -> Frame Conversion2/1
  Frame Conversion1/1 -> AudioOut/1
  Frame Conversion2/1 -> SampleRateConverter/1

== system ModelDemopalooza/PreAmp/SrcUp ==
  AudioIn : Inport
  Frame Conversion : FrameConversion
  Frame Conversion1 : FrameConversion  OutFrame=Sample-based
  SampleRateConverter1 : SampleRateConverter/SampleRateConverter  UPFACTOR=13  DOWNFACTOR=12  OUTFRAME_SIZE=-1  RATE_SELECTOR=Input Sample Rate  FS=48000  FPASSBAND=16500  FHEARING=19000  PASSBAND_RIPPLE=60  STOPBAND_ATTENUATION=60
  AudioOut : Outport
  wires:
  SampleRateConverter1/1 -> Frame Conversion1/1
  Frame Conversion/1 -> SampleRateConverter1/1
  Frame Conversion1/1 -> AudioOut/1
  AudioIn/1 -> Frame Conversion/1

== system ModelDemopalooza/PostProcess/PostProcess/EnergyLimiter ==
  In1 : Inport
  EnergyLimiter : EnergyLimiter/EnergyLimiter  EnableGainLimiter=EnableGainLimiter  EnergyMeasurementTimeConstantInSeconds=EnergyMeasurementTimeConstantInSeconds  GainChangeStepIndB=GainChangeStepIndB  MaxEnergyLevelIndB=MaxEnergyLevelIndB  EnergyAdjustmentFactorIndB=EnergyAdjustmentFactorIndB  MaxChannels=MaxChannels  GainIncreaseDurationInSeconds=GainIncreaseDurationInSeconds  GainDecreaseDurationInSeconds=GainDecreaseDurationInSeconds  MaxGainReductionIndB=MaxGainReductionIndB  sample_rate_in_hertz=sample_rate_in_hertz  frameSize=frameSize  CurrentGainVal=CurrentGainVal
  Terminator : Terminator
  Out1 : Outport
  wires:
  EnergyLimiter/2 -> Terminator/1
  In1/1 -> EnergyLimiter/1
  EnergyLimiter/1 -> Out1/1

== system ModelDemopalooza/PostProcess/PostProcess/Limiter ==
  In1 : Inport
  Terminator : Terminator
  limiter : Limiter/Limiter  attackDB=10e3 * ones(1,sys_defs.number_of_output_audio_channels)  decayDB=100 * ones(1,sys_defs.number_of_output_audio_channels)  maxAttackTuningValue=10 * ones(1,sys_defs.number_of_output_audio_channels)  threshold=0.9 * ones(1,sys_defs.number_of_output_audio_channels)  attackDB_low=10e3 * ones(1,sys_defs.number_of_output_audio_channels)  decayDB_low=100 * ones(1,sys_defs.number_of_output_audio_channels)  maxAttack_low=10 * ones(1,sys_defs.number_of_output_audio_channels)  threshold_low=0.9 * ones(1,sys_defs.number_of_output_audio_channels)
  Out1 : Outport  VectorParamsAs1DForOutWhenUnconnected=off
  wires:
  In1/1 -> limiter/1
  limiter/1 -> Out1/1
  [EntLimiterSoftclipParamSet] -> limiter/2
  [EntLimiterSoftclipDisableMsg] -> limiter/3
  limiter/2 -> Terminator/1

== system ModelDemopalooza/PostProcess/PostProcess/Mute ==
  In1 : Inport
  mute : Mute/mute  initial_mute_state=ent_mute_init  samplesPerFrame=32  MaskFeatureName=Mute
  Out1 : Outport  VectorParamsAs1DForOutWhenUnconnected=off
  wires:
  In1/1 -> mute/1
  mute/1 -> Out1/1

== system ModelDemopalooza/PostProcess/PostProcess/OutputEQ ==
  In1 : Inport
  Pooliir with Non-Trivial Translations : PooliirLib/PooliirwithNonTrivialTranslations  maxNumStages=64  numStages=outputEQ.numStages  sosCoefficients=outputEQ.coeffs  FeatureName=EQ
  Out1 : Outport
  wires:
  Pooliir with Non-Trivial Translations/1 -> Out1/1
  In1/1 -> Pooliir with Non-Trivial Translations/1

== system ModelDemopalooza/PostProcess/PostProcess/Soft Clipper ==
  In1 : Inport
  Terminator : Terminator
  soft clipper : Softclipper/SoftClipper  MaxXminLow=0.65  MaskXmin=0.65  MaskYMax=1  MaskYMaxLow=1
  Out1 : Outport  VectorParamsAs1DForOutWhenUnconnected=off
  wires:
  In1/1 -> soft clipper/1
  soft clipper/1 -> Out1/1
  [EntLimiterSoftclipParamSet] -> soft clipper/2
  [EntLimiterSoftclipDisableMsg] -> soft clipper/3
  soft clipper/2 -> Terminator/1

== system ModelDemopalooza/PreAmp/DecRate/AudioPilot35 ==
  MusicIn : Inport
  Mic : Inport  Port=2
  PreVolumeAudio : Inport  Port=3
  VolumeGain : Inport  Port=4
  LFRef : Inport  Port=5
  HFRefLPF : Inport  Port=6
  AnnTrigger : Inport  Port=7
  Audiopilot_3_5 : Audiopilot_3_5/Audiopilot_3_5  FeatureName=Audiopilot  InputAudioMode=Stereo - 2 Channels  NoiseEstimationMode=Regular  IncludeSpumTails=off  IncludeIgnoreMicFlag=off  Config=[]
  Delay1 : Delay  DelayLength=32
  Delay2 : Delay  DelayLength=32
  EntertainmentLevelDetection : EntertainmentLevelDetection/EntertainmentLevelDetection  NumInputChannels=AUDIOPILOT_NUM_MUSIC_IN  FANEnable=off  BODEnable=off  Config=[]
  Terminator : Terminator
  MusicOut : Outport
  WBNoisedbspl : Outport  Port=2
  wires:
  PreVolumeAudio/1 -> EntertainmentLevelDetection/1
  AnnTrigger/1 -> EntertainmentLevelDetection/3
  EntertainmentLevelDetection/1 -> Terminator/1
  VolumeGain/1 -> EntertainmentLevelDetection/2
  LFRef/1 -> Delay1/1
  Audiopilot_3_5/2 -> WBNoisedbspl/1
  HFRefLPF/1 -> Delay2/1
  Audiopilot_3_5/1 -> MusicOut/1
  MusicIn/1 -> Audiopilot_3_5/1
  Mic/1 -> Audiopilot_3_5/2
  Delay1/1 -> Audiopilot_3_5/3
  Delay2/1 -> Audiopilot_3_5/4
  EntertainmentLevelDetection/2 -> Audiopilot_3_5/5
  EntertainmentLevelDetection/3 -> Audiopilot_3_5/6

== system ModelDemopalooza/PreAmp/DecRate/Medusa5H1 ==
  AudioIn : Inport
  AnnNonHeadrestDR : Inport  Port=2
  AnnHeadrestDR : Inport  Port=3
  AnnFR : Inport  Port=4
  AnnEnable : Inport  Port=5
  Balance : Subsystem
  MedusaHoligram : Subsystem  AncestorBlock=medusa5h1_stereo/Medusa + Holigram  mask{config=MedusaConfig, vlsConfigStruct=VLSConfig}
      mask prompts: config "Medusa config struct name:"; vlsConfigStruct "VLS config struct name:"
      mask init:
      | tailCompEQ = config.tailCompEQ;
      | HRDelayConfig = vlsConfigStruct.HeadrestDelayConfig;
      settings: LibrarySourceBlock=medusa5h1_stereo/Medusa + Holigram
  MedusaPostHoligram : Subsystem
  PreAmpPart2 : Subsystem
  VLS : VLS/VLS  configStruct=VLSConfig
  AudioOut : Outport
  LFRef : Outport  Port=2
  HFRef : Outport  Port=3
  wires:
  MedusaHoligram/6(HFRef) -> HFRef/1
  MedusaHoligram/2(P gains) -> VLS/4
  MedusaHoligram/1(D gains) -> VLS/3
  MedusaHoligram/5(LFRef) -> LFRef/1
  AudioIn/1 -> Balance/1(In)
  Balance/1(Out) -> MedusaHoligram/1(AudioIn)
  AnnEnable/1 -> ?
  AnnHeadrestDR/1 -> VLS/2
  MedusaHoligram/3(DROut) -> PreAmpPart2/1(DR)
  MedusaHoligram/4(FROut) -> PreAmpPart2/2(FR)
  PreAmpPart2/1(DRHeadrestComps) -> [VlsIn]
  PreAmpPart2/4(FadeGains) -> MedusaHoligram/2(FadeIn)
  AnnNonHeadrestDR/1 -> MedusaPostHoligram/4(AnnNonHeadresrDR)
  AnnFR/1 -> MedusaPostHoligram/5(AnnFR)
  VLS/1 -> MedusaPostHoligram/1(HeadrestDRIn)
  MedusaPostHoligram/1(AudioOut) -> AudioOut/1
  PreAmpPart2/2(DRNonHeadrestSpkr) -> MedusaPostHoligram/2(NonHeadrestDRIn)
  PreAmpPart2/3(FRSpkr) -> MedusaPostHoligram/3(FRIn)
  [VlsIn] -> VLS/1

== system ModelDemopalooza/PreAmp/DecRate/Medusa5H1/Balance ==
  In : Inport
  Balance : BalanceBtc/Balance  FeatureName=Balance  Config=Balance
      settings: SourceProductName=Bose Blocklib
  Out : Outport
  wires:
  Balance/1 -> Out/1
  In/1 -> Balance/1

== system ModelDemopalooza/PreAmp/DecRate/Medusa5H1/MedusaHoligram ==
  AudioIn : Inport
  FadeIn : Inport  Port=2  OutDataTypeStr=single
  FeaturePath : FeaturePath/FeaturePath  FeatureName=Medusa  IsGroup=off  GroupNumber=-1  IsModule=off  TriggerInit=[90 69 205 176]
      settings: SourceProductName=Bose Talaria
  Medusa5H1 Part 1 : Subsystem  TreatAsAtomicUnit=on
      settings: RTWSystemCode=Nonreusable function
  Medusa5H1 Part 2 : Subsystem  TreatAsAtomicUnit=on
      settings: RTWSystemCode=Nonreusable function
  Medusa5H1 Part 3 : Subsystem  TreatAsAtomicUnit=on
      settings: RTWSystemCode=Nonreusable function  FunctionWithSeparateData=on
  Medusa5H1 Part 4 : Subsystem  TreatAsAtomicUnit=on  RTWFcnName=MedusaHoligram  RTWFileName=MedusaHoligram
      settings: RTWSystemCode=Nonreusable function  RTWFcnNameOpts=User specified  RTWFileNameOpts=User specified  FunctionWithSeparateData=on
  Medusa5H1 Part 5 : Subsystem  TreatAsAtomicUnit=on
      settings: RTWSystemCode=Nonreusable function  FunctionWithSeparateData=on
  D gains : Outport
  P gains : Outport  Port=2
  DROut : Outport  Port=3
  FROut : Outport  Port=4
  LFRef : Outport  Port=5  VectorParamsAs1DForOutWhenUnconnected=off
  HFRef : Outport  Port=6  VectorParamsAs1DForOutWhenUnconnected=off
  wires:
  Medusa5H1 Part 1/4(CAEEnable) -> Medusa5H1 Part 2/4(CAEEnable)
  Medusa5H1 Part 2/3(HFRef) -> HFRef/1
  Medusa5H1 Part 5/2(FROut) -> FROut/1
  Medusa5H1 Part 5/1(DROut) -> DROut/1
  Medusa5H1 Part 4/2(FROut) -> Medusa5H1 Part 5/2(FRIn)
  Medusa5H1 Part 4/1(DROut) -> Medusa5H1 Part 5/1(DRIn)
  Medusa5H1 Part 3/1(D gains) -> D gains/1
  Medusa5H1 Part 3/3(HeadrestPremixOut) -> Medusa5H1 Part 4/1(HeadrestComps)
  Medusa5H1 Part 3/2(P gains) -> P gains/1
  Medusa5H1 Part 3/4(NonHeadrestPremixOut) -> Medusa5H1 Part 4/2(NonHeadrestComps)
  Medusa5H1 Part 1/1(LRbass) -> Medusa5H1 Part 3/1(Bass)
  [AudioIn] -> Medusa5H1 Part 2/1(AudioIn)
  Medusa5H1 Part 1/2(LRbp) -> Medusa5H1 Part 2/2(LRbp)
  Medusa5H1 Part 1/3(LRhp) -> Medusa5H1 Part 2/3(LRhp)
  Medusa5H1 Part 1/5(Mono) -> LFRef/1
  AudioIn/1 -> Medusa5H1 Part 1/1(AudioIn), [AudioIn]
  FadeIn/1 -> Medusa5H1 Part 3/4(FadeIn)
  Medusa5H1 Part 3/5(FRMixerOut) -> Medusa5H1 Part 4/3(FRSpkr)
  Medusa5H1 Part 2/1(DRComps) -> Medusa5H1 Part 3/2(DRComps)
  Medusa5H1 Part 2/2(FRComps) -> Medusa5H1 Part 3/3(FRComps)

== system ModelDemopalooza/PreAmp/DecRate/Medusa5H1/MedusaPostHoligram ==
  HeadrestDRIn : Inport
  NonHeadrestDRIn : Inport  Port=2
  FRIn : Inport  Port=3
  AnnNonHeadresrDR : Inport  Port=4
  AnnFR : Inport  Port=5
  Add : Sum
  Add1 : Sum
  MedusaPostHoligram : medusa5h1_stereo/Medusa Post Holigram  config=MedusaConfig
  AudioOut : Outport
  wires:
  HeadrestDRIn/1 -> MedusaPostHoligram/1
  MedusaPostHoligram/1 -> AudioOut/1
  NonHeadrestDRIn/1 -> Add/1
  AnnNonHeadresrDR/1 -> Add/2
  Add/1 -> MedusaPostHoligram/2
  FRIn/1 -> Add1/1
  Add1/1 -> MedusaPostHoligram/3
  AnnFR/1 -> Add1/2

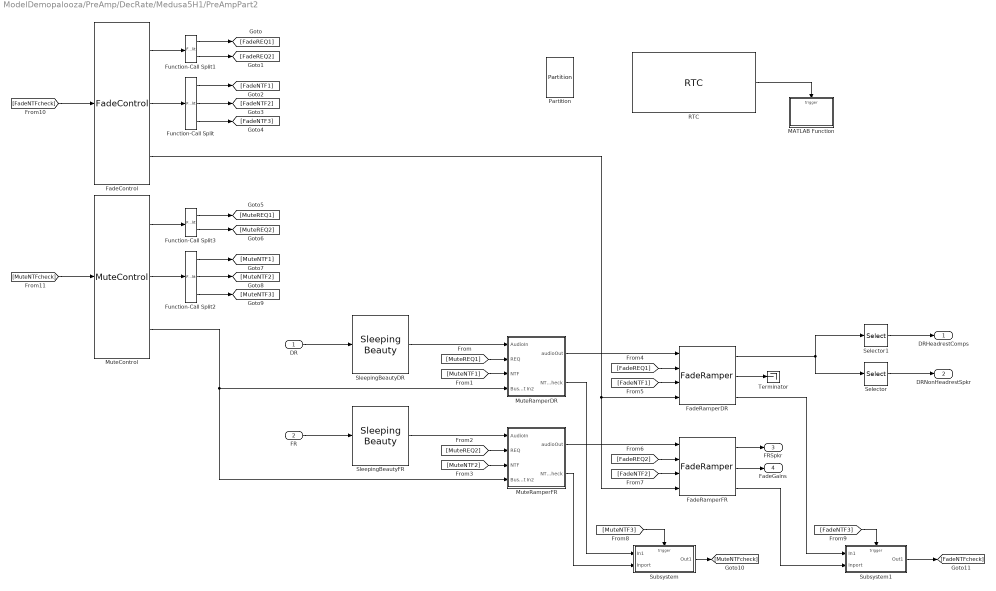
== system ModelDemopalooza/PreAmp/DecRate/Medusa5H1/PreAmpPart2 ==
  DR : Inport
  FR : Inport  Port=2
  FadeControl : FadeControl/FadeControl  BankNumber=0  MaskIndexOffset=128  MaskBoostDisable=off  MaskSilentExtreme=on
  FadeRamperDR : FadeRamper/FadeRamper  MaskFeatureName=FadeRamperDR  MaskChanRampMap=ones(1,30)  MaskEnableGainPort=on
  FadeRamperFR : FadeRamper/FadeRamper  MaskFeatureName=FadeRamperFR  MaskChanRampMap=ones(1,22)  MaskEnableGainPort=on
  Function-Call Split : FunctionCallSplit  IconShape=distinctive  NumOutputPorts=3  OutputPortLayout=default
  Function-Call Split1 : FunctionCallSplit  IconShape=distinctive  NumOutputPorts=2  OutputPortLayout=default
  Function-Call Split2 : FunctionCallSplit  IconShape=distinctive  NumOutputPorts=3  OutputPortLayout=default
  Function-Call Split3 : FunctionCallSplit  IconShape=distinctive  NumOutputPorts=2  OutputPortLayout=default
  MATLAB Function : MATLAB Function  TreatAsAtomicUnit=on
  MuteControl : MuteControl/MuteControl
  MuteRamperDR : Subsystem  AncestorBlock=MuteRamper/MuteRamper  mask(Bose MuteRamper){initial_mute_state=0, samplesPerFrame=8}
      mask prompts: initial_mute_state "Initially muted (logical)"; samplesPerFrame "Samples per Frame"
      mask help: This component is to be used in conjunction with the MuteControl block, which provides runtime control and tuning capabilities via an RTC and the tune variable muteControlRampTime. Multiple instances of this block may be placed within an audio application, and a single MuteControl block has the ability to control all of these rampers simultaneously.
      mask init:
      | blkh = gcbh;
      | % Copy discrete mask parameters into a classdef object
      | InnerLinkConfig = MuteRamperConfig;
      | InnerLinkConfig.InitialMuteState = initial_mute_state;
      | InnerLinkConfig.SamplesPerFrame = samplesPerFrame;
      settings: LibrarySourceBlock=MuteRamper/MuteRamper
  MuteRamperFR : Subsystem  AncestorBlock=MuteRamper/MuteRamper  mask(Bose MuteRamper){initial_mute_state=0, samplesPerFrame=32}
      mask prompts: initial_mute_state "Initially muted (logical)"; samplesPerFrame "Samples per Frame"
      mask help: This component is to be used in conjunction with the MuteControl block, which provides runtime control and tuning capabilities via an RTC and the tune variable muteControlRampTime. Multiple instances of this block may be placed within an audio application, and a single MuteControl block has the ability to control all of these rampers simultaneously.
      mask init: same as ModelDemopalooza/PreAmp/DecRate/Medusa5H1/PreAmpPart2/MuteRamperDR
      settings: LibrarySourceBlock=MuteRamper/MuteRamper
  Partition : FeaturePath/Partition  PartitionNumber=1  TriggerInit=[635 -229 680 -161]
      settings: SourceProductName=Bose Talaria
  RTC : RTC/RTC  REQ_Priority=RTC_Mask.NormalPriority  RequestAtInit=off  EnableRequest=on  REQElemType1=uint32  REQElemWidth1=1  REQElemInitial1=[]  REQElemType2=uint32  REQElemWidth2=1  REQElemInitial2=[]  REQElemType3=uint32  REQElemWidth3=1  REQElemInitial3=[]  REQElemType4=uint32  REQElemWidth4=1  REQElemInitial4=[]  REQElemType5=uint32  REQElemWidth5=1  REQElemInitial5=[]  REQElemType6=uint32  REQElemWidth6=1  REQElemInitial6=[]  REQElemType7=uint32  REQElemWidth7=1  REQElemInitial7=[]  REQElemType8=uint32  REQElemWidth8=1  REQElemInitial8=[]  REQElemType9=uint32  REQElemWidth9=1  REQElemInitial9=[]  REQElemType10=uint32  REQElemWidth10=1  REQElemInitial10=[]  EnableResponse=on  EnableRSP_StatusIn=off  RSPElemType1=uint32  RSPElemWidth1=1  RSPElemType2=uint32  RSPElemWidth2=1  RSPElemType3=uint32  RSPElemWidth3=1  RSPElemType4=uint32  RSPElemWidth4=1  RSPElemType5=uint32  RSPElemWidth5=1  RSPElemType6=uint32  RSPElemWidth6=1  RSPElemType7=uint32  RSPElemWidth7=1  RSPElemType8=uint32  RSPElemWidth8=1  RSPElemType9=uint32  RSPElemWidth9=1  RSPElemType10=uint32  RSPElemWidth10=1  EnableNotification=off  EnableNTF_PrepTrig=off  NTFElemType1=uint32  NTFElemWidth1=1  NTFElemType2=uint32  NTFElemWidth2=1  NTFElemType3=uint32  NTFElemWidth3=1  NTFElemType4=uint32  NTFElemWidth4=1  NTFElemType5=uint32  NTFElemWidth5=1  NTFElemType6=uint32  NTFElemWidth6=1  NTFElemType7=uint32  NTFElemWidth7=1  NTFElemType8=uint32  NTFElemWidth8=1  NTFElemType9=uint32  NTFElemWidth9=1  NTFElemType10=uint32  NTFElemWidth10=1  MaskMessageName=ResetSleepingBeauty
      settings: SourceProductName=Bose Talaria
  Selector : Selector  NumberOfDimensions=2  InputPortWidth=3  IndexOptions=Select all,Index vector (dialog)  Indices=[1 3],1:MedusaConfig.numNonHeadrest  OutputSizes=1,1
  Selector1 : Selector  NumberOfDimensions=2  InputPortWidth=3  IndexOptions=Select all,Index vector (dialog)  Indices=[1 3],MedusaConfig.numNonHeadrest+1:MedusaConfig.numDRChan  OutputSizes=1,1
  SleepingBeautyDR : SleepingBeauty/Sleeping Beauty  MaskFeatureName=SleepingBeautyDR  MaskChanRampMap=ones(1,30)  MaskOffset=128  MaskSilentExtremeMutesBass=off
  SleepingBeautyFR : SleepingBeauty/Sleeping Beauty  MaskFeatureName=SleepingBeautyFR  MaskChanRampMap=ones(1,22)  MaskOffset=128  MaskSilentExtremeMutesBass=off
  Subsystem : Subsystem
  Subsystem1 : Subsystem
  Terminator : Terminator
  DRHeadrestComps : Outport
  DRNonHeadrestSpkr : Outport  Port=2
  FRSpkr : Outport  Port=3
  FadeGains : Outport  Port=4
  wires:
  Function-Call Split2/3 -> [MuteNTF3]
  [FadeNTF1] -> FadeRamperDR/3
  FR/1 -> SleepingBeautyFR/1
  Function-Call Split2/2 -> [MuteNTF2]
  Function-Call Split3/2 -> [MuteREQ2]
  MuteControl/2 -> Function-Call Split2/1
  [FadeREQ2] -> FadeRamperFR/2
  Function-Call Split1/2 -> [FadeREQ2]
  FadeControl/2 -> Function-Call Split/1
  [FadeNTF3] -> Subsystem1/Trigger
  Function-Call Split1/1 -> [FadeREQ1]
  [MuteREQ2] -> MuteRamperFR/2(REQ)
  [MuteNTF3] -> Subsystem/Trigger
  [MuteNTF1] -> MuteRamperDR/3(NTF)
  [FadeNTF2] -> FadeRamperFR/3
  FadeControl/1 -> Function-Call Split1/1
  [FadeNTFcheck] -> FadeControl/1
  MuteRamperDR/1(audioOut) -> FadeRamperDR/1
  [MuteREQ1] -> MuteRamperDR/2(REQ)
  Function-Call Split2/1 -> [MuteNTF1]
  Function-Call Split3/1 -> [MuteREQ1]
  SleepingBeautyDR/1 -> MuteRamperDR/1(AudioIn)
  RTC/1 -> MATLAB Function/Trigger
  FadeRamperDR/2 -> Terminator/1
  Selector1/1 -> DRHeadrestComps/1
  MuteRamperFR/2(NTF_check) -> Subsystem/2(Inport)
  Selector/1 -> DRNonHeadrestSpkr/1
  Subsystem/1(Out1) -> [MuteNTFcheck]
  [MuteNTFcheck] -> MuteControl/1
  [FadeREQ1] -> FadeRamperDR/2
  [MuteNTF2] -> MuteRamperFR/3(NTF)
  MuteControl/1 -> Function-Call Split3/1
  Function-Call Split/2 -> [FadeNTF2]
  FadeRamperDR/3 -> Subsystem1/1(In1)
  FadeRamperFR/2 -> FadeGains/1
  Subsystem1/1(Out1) -> [FadeNTFcheck]
  FadeRamperFR/3 -> Subsystem1/2(Inport)
  SleepingBeautyFR/1 -> MuteRamperFR/1(AudioIn)
  DR/1 -> SleepingBeautyDR/1
  MuteRamperDR/2(NTF_check) -> Subsystem/1(In1)
  FadeRamperFR/1 -> FRSpkr/1
  Function-Call Split/3 -> [FadeNTF3]
  FadeRamperDR/1 -> Selector1/1, Selector/1
  MuteControl/3 -> MuteRamperFR/4(Bus Element In2), MuteRamperDR/4(Bus Element In2)
  Function-Call Split/1 -> [FadeNTF1]
  MuteRamperFR/1(audioOut) -> FadeRamperFR/1
  FadeControl/3 -> FadeRamperFR/4, FadeRamperDR/4

== system ModelDemopalooza/PreAmp/DecRate/Medusa5H1/MedusaHoligram/Medusa5H1 Part 1 ==
  AudioIn : Inport
  Bass Manager Stereo : BassManager/MedusaBassManagerStereo  Config=Config.BassManager
  CAE Treble Boost : Subsystem  Variant=on
  Mean : dspstat3/Mean  run=off  InputProcessing=Columns as channels (frame based)  reset_popup=None  directionMode=Each row  dimension=1  roiEnable=off  roiType=Rectangles  roiPortion=Entire ROI  roiOutput=Individual statistics for each ROI  roiFlag=off  roundingMode=Floor  overflowMode=off  outputDataTypeStr=Inherit: Same as accumulator  outputMin=[]  outputMax=[]  outputLastDataTypeStr=Inherit: Same as accumulator
  Medusa Band Split Stereo : Subsystem  AncestorBlock=MedusaBandSplit/Medusa Band Split Stereo  mask(Medusa Band Split Stereo){configStruct=config.BandSplitConfig, numInputs=2}
      mask prompts: configStruct "Config struct name:"; numInputs "Number of inputs:"
      mask help:
      | This block performs bandsplitting and downsampling for stereo inputs used by Medusa system.
      |
      | Configuration struct needs to define the below fields with the exact names which are used inside the block.
      |
      | D: Decimation factor
      | ifir: Interpolated filter coefficients
      | fireven: Image rejection filter coefficients
      | upfir: Reconstruction filter coefficients
      | band_separation_delay: Alignment delay for the whole Bandsplit
      |
      | For more information and sample generation of config struct, please see 'Help'.
      settings: LibrarySourceBlock=MedusaBandSplit/Medusa Band Split Stereo
      mask Help:
      | Model that uses Band Split block need to call <i>MedusaBandSplitInit()</i> to generate <i>MedusaBandSplitConfig</i> in base workspace.
      | 
      | <b>Sample usage:</b>
      | 
      | MedusaConfig = generateMedusaConfig(auto_gen_sys_defs);
      | MedusaBandSplitInit(MedusaConfig);
      | or
      | DefaultMedusaConfig = generateMedusaConfig();
      | MedusaBandSplitInit(DefaultMedusaConfig);
  Partition : FeaturePath/Partition  PartitionNumber=2  TriggerInit=[375 -99 420 -31]
      settings: SourceProductName=Bose Talaria
  LRbass : Outport  VectorParamsAs1DForOutWhenUnconnected=off
  LRbp : Outport  Port=2  VectorParamsAs1DForOutWhenUnconnected=off
  LRhp : Outport  Port=3  VectorParamsAs1DForOutWhenUnconnected=off
  CAEEnable : Outport  Port=4
  Mono : Outport  Port=5  VectorParamsAs1DForOutWhenUnconnected=off
  wires:
  CAE Treble Boost/2(CAEEnable) -> CAEEnable/1
  AudioIn/1 -> CAE Treble Boost/1(AudioIn)  "L, R"
  Mean/1 -> Mono/1
  CAE Treble Boost/1(Out) -> Bass Manager Stereo/1, Mean/1  "L, R"
  Bass Manager Stereo/2 -> Medusa Band Split Stereo/1(LRhp)
  Medusa Band Split Stereo/1(LRbp) -> LRbp/1  "LRbp"
  Bass Manager Stereo/1 -> LRbass/1  "Lbass, Rbass"
  Medusa Band Split Stereo/2(LRtreble) -> LRhp/1  "LRtreble"
